simulink library "relay_mgc_cmd_lib"  (Simulink 8.1)
settings: Solver=ode45  StartTime=0.0  StopTime=10.0  RelTol=1e-3
undefined symbols (not defined in the file or in its folder): relay_settings
libraries: simulink x1
settings Model: Creator=RE25624  LastModifiedBy=re25624

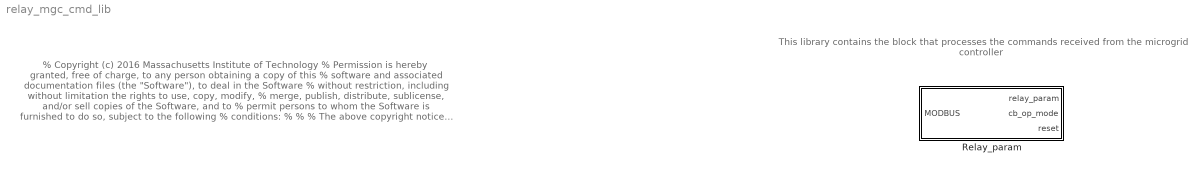
== system relay_mgc_cmd_lib ==
  note: This library contains the block that processes the commands
      | received from the microgrid controller
  note: % Copyright (c) 2016 Massachusetts Institute of Technology
      | % Permission is hereby granted, free of charge, to any person obtaining a copy of this
      | % software and associated documentation files (the "Software"), to deal in the Software
      | % without restriction, including without limitation the rights to use, copy, modify,
      | % merge, publish, distribute, sublicense, and/or sell copies of the Software, and to
      | % permit persons to whom the Software is furnished to do so, subject to the following
      | % conditions:
      | %
      | %
      | % The above copyright notice and this permission notice shall be included in
      | % all copies or substantial portions of the Software.
      | %
      | % THE SOFTWARE IS PROVIDED "AS IS", WITHOUT WARRANTY OF ANY KIND, EXPRESS OR IMPLIED,
      | % INCLUDING BUT NOT LIMITED TO THE WARRANTIES OF MERCHANTABILITY, FITNESS FOR A
      | % PARTICULAR PURPOSE AND NONINFRINGEMENT. IN NO EVENT SHALL THE AUTHORS OR COPYRIGHT
      | % HOLDERS BE LIABLE FOR ANY CLAIM, DAMAGES OR OTHER LIABILITY, WHETHER IN AN ACTION
      | % OF CONTRACT, TORT OR OTHERWISE, ARISING FROM, OUT OF OR IN CONNECTION WITH THE
      | % SOFTWARE OR THE USE OR OTHER DEALINGS IN THE SOFTWARE.
      | %
      | %
      | %%
  Relay_param : Subsystem  mask(MGC Commands through MODBUS){relay_settings=relay_settings}
      mask prompts: relay_settings "Relay Settings"
      mask help:
      | 0) This block receives the commands from the microgrid controller through MODBUS
      | 1) This block facilitates the application of two independent sets of protection settings to the relays
      | 2) protection_mode = 0 selects the first group of settings (default) --- settings most be defined in the workspace (currently done using excel files)
      | 3) protection_mode = 1 selects the second group of settings --- settings most be defined in the workspace (currently done using excel files)
      | 4) This block permits the microgrid controller to select the protection modes during the simulation
      | 5) If no signal is received from the microgrid, the protection_mode variable will default to "0" which corresponds to group#1 parameters
      |
      |
      | Procedure to reclose a breaker:
      | 1) reset all relay functions
      | 2) set cb_op_mode==1 to force breaker to close
      |    --> The relay function 25 will automatically activate
      | 3) change cb_op_mode==0 for logic based operation
      |
      | Required relay settings:
      | 1.  Relay#
      | 2.  Nominal VRMSLL
      | 3.  Max. Slip Voltage [%]
      | 4.  Max. Slip Angle [degree]
      | 5.  Max. Slip Frequency [Hz]
      | 6.  27P and 59P Trip Delay [Sec]
      | 7.  CT Ratio
      | 8.  50P IOC Trip Pickup [amp sec]
      | 9.  50P IOC Trip Delay [sec]
      | 10.  51P TOC Trip Pickup [amp sec]
      | 11.  51P Curve
      | 12.  51P TOC Time Dial
      | 13.  27P Trip Pickup [pu]
      | 14.  59P Trip Pickup [pu]
      | 15.  50P IOC Trip Pickup [amp sec]
      | 16.  50P IOC Trip Delay [sec]
      | 17.  51P TOC Trip Pickup [amp sec]
      | 18.  51P Curve
      | 19.  51P TOC Time Dial
      | 20.  27P Trip Pickup [pu]
      | 21.  59P Trip Pickup [pu]

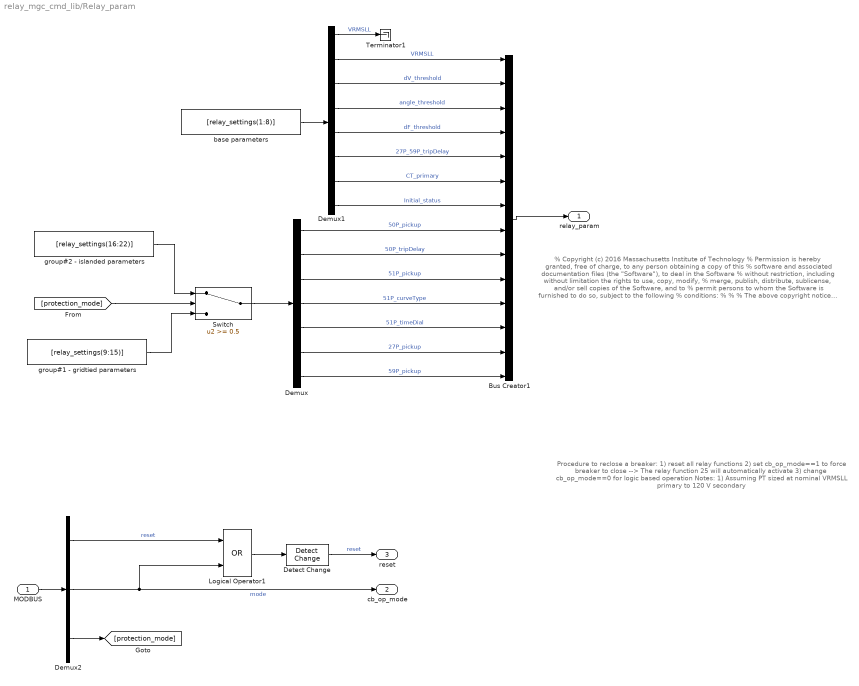
== system relay_mgc_cmd_lib/Relay_param ==
  note: Procedure to reclose a breaker:
      | 1) reset all relay functions
      | 2) set cb_op_mode==1 to force breaker to close
      |    --> The relay function 25 will automatically activate
      | 3) change cb_op_mode==0 for logic based operation
      |
      |
      | Notes:
      | 1) Assuming PT sized at nominal VRMSLL primary to 120 V secondary
  note: % Copyright (c) 2016 Massachusetts Institute of Technology
      | % Permission is hereby granted, free of charge, to any person obtaining a copy of this
      | % software and associated documentation files (the "Software"), to deal in the Software
      | % without restriction, including without limitation the rights to use, copy, modify,
      | % merge, publish, distribute, sublicense, and/or sell copies of the Software, and to
      | % permit persons to whom the Software is furnished to do so, subject to the following
      | % conditions:
      | %
      | %
      | % The above copyright notice and this permission notice shall be included in
      | % all copies or substantial portions of the Software.
      | %
      | % THE SOFTWARE IS PROVIDED "AS IS", WITHOUT WARRANTY OF ANY KIND, EXPRESS OR IMPLIED,
      | % INCLUDING BUT NOT LIMITED TO THE WARRANTIES OF MERCHANTABILITY, FITNESS FOR A
      | % PARTICULAR PURPOSE AND NONINFRINGEMENT. IN NO EVENT SHALL THE AUTHORS OR COPYRIGHT
      | % HOLDERS BE LIABLE FOR ANY CLAIM, DAMAGES OR OTHER LIABILITY, WHETHER IN AN ACTION
      | % OF CONTRACT, TORT OR OTHERWISE, ARISING FROM, OUT OF OR IN CONNECTION WITH THE
      | % SOFTWARE OR THE USE OR OTHER DEALINGS IN THE SOFTWARE.
      | %
      | %
      | %%
  MODBUS : Inport
  Bus Creator1 : BusCreator  Inputs=14
  Demux : Demux  Outputs=7
  Demux1 : Demux  Outputs=8
  Demux2 : Demux  Outputs=3
  Detect Change : simulink/Logic and Bit Operations/Detect Change  vinit=0  InputProcessing=Inherited  OutDataTypeStr=uint8
  Logical Operator1 : Logic  Operator=OR  AllPortsSameDT=off  OutDataTypeStr=boolean
  Switch : Switch  Threshold=0.5
  Terminator1 : Terminator
  base parameters : Constant  Value=[relay_settings(1:8)]
  group#1 - gridtied parameters : Constant  Value=[relay_settings(9:15)]
  group#2 - islanded parameters : Constant  Value=[relay_settings(16:22)]
  relay_param : Outport
  cb_op_mode : Outport  Port=2
  reset : Outport  Port=3
  wires:
  Demux2/3 -> [protection_mode]
  Demux2/2 -> cb_op_mode/1, Logical Operator1/2  "mode"
  MODBUS/1 -> Demux2/1
  Demux2/1 -> Logical Operator1/1  "reset"
  Logical Operator1/1 -> Detect Change/1
  Detect Change/1 -> reset/1  "reset"
  Switch/1 -> Demux/1
  base parameters/1 -> Demux1/1
  Demux1/1 -> Terminator1/1  "VRMSLL"
  [protection_mode] -> Switch/2
  Bus Creator1/1 -> relay_param/1
  group#1 - gridtied parameters/1 -> Switch/3
  group#2 - islanded parameters/1 -> Switch/1
  Demux1/6 -> Bus Creator1/5  "27P_59P_tripDelay"
  Demux1/7 -> Bus Creator1/6  "CT_primary"
  Demux1/5 -> Bus Creator1/4  "dF_threshold"
  Demux1/4 -> Bus Creator1/3  "angle_threshold"
  Demux1/8 -> Bus Creator1/7  "Initial_status"
  Demux1/3 -> Bus Creator1/2  "dV_threshold"
  Demux1/2 -> Bus Creator1/1  "VRMSLL"
  Demux/5 -> Bus Creator1/12  "51P_timeDial"
  Demux/4 -> Bus Creator1/11  "51P_curveType"
  Demux/2 -> Bus Creator1/9  "50P_tripDelay"
  Demux/1 -> Bus Creator1/8  "50P_pickup"
  Demux/7 -> Bus Creator1/14  "59P_pickup"
  Demux/6 -> Bus Creator1/13  "27P_pickup"
  Demux/3 -> Bus Creator1/10  "51P_pickup"
